simulink model "mavsim_chap8"  (R2015a)
settings: Solver=ode15s  StartTime=0.0  StopTime=80  RelTol=1e-3
InitFcn:
  | param_chap8
undefined symbols (not defined in the file or in its folder): autopilot, drawAircraft, estimate_states, forces_moments, gps, P, plotextramavstatevariables, plotmavstatevariables, sensors, true_states
libraries: simulink x4
settings Model: CovSFcnEnable=off  Creator=beard  LastModifiedBy=Scott
settings DataIOCC: SignalLoggingSaveFormat=ModelDataLogs
settings OptimizationCC: ExpressionDepthLimit=2147483647  InitFltsAndDblsToZero=on
settings DebuggingCC: UnderspecifiedInitializationDetection=Classic  MergeDetectMultiDrivingBlocksExec=none  SolverPrmCheckMsg=warning  FcnCallInpInsideContextMsg=UseLocalSettings  StateNameClashWarn=warning
settings SFSimCC: SimParseCustomCode=off
settings GRTTargetCC: CombineOutputUpdateFcns=off  GRTInterface=on

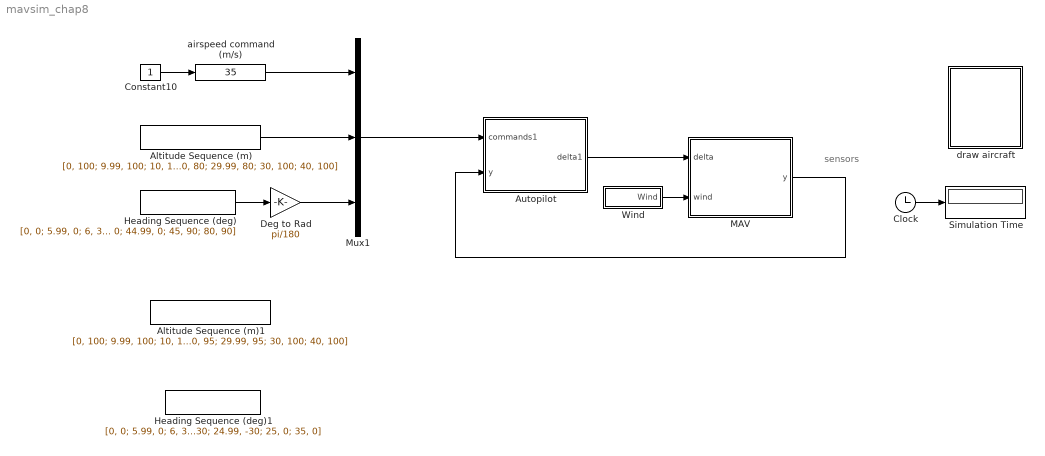
== system mavsim_chap8 ==
  note: sensors
  Altitude Sequence (m) : FromWorkspace  VariableName=[0, 100; 9.99, 100; 10, 120; 19.99, 120; 20, 80; 29.99, 80; 30, 100; 40, 100]  SampleTime=0
  Altitude Sequence (m)1 : FromWorkspace  VariableName=[0, 100; 9.99, 100; 10, 105; 19.99, 105; 20, 95; 29.99, 95; 30, 100; 40, 100]  SampleTime=0
  Autopilot : Subsystem
      mask Display: image(imread('kestrel.jpg'))
  Clock : Clock
  Constant10 : Constant
  Deg to Rad : Gain  Gain=pi/180
  Heading Sequence (deg) : FromWorkspace  VariableName=[0, 0; 5.99, 0; 6, 30; 14.99, 30; 15, -30; 24.99, -30; 25, 0; 35, 0; 44.99, 0; 45, 90; 80, 90]  SampleTime=0
  Heading Sequence (deg)1 : FromWorkspace  VariableName=[0, 0; 5.99, 0; 6, 30; 14.99, 30; 15, -30; 24.99, -30; 25, 0; 35, 0]  SampleTime=0
  MAV : Subsystem
      mask Display: image(imread('batcam.png'))
  Mux1 : Mux  Inputs=3
  Simulation Time : Display
  Wind : Subsystem
  airspeed command (m/s) : simulink/Math Operations/Slider Gain  low=5  gain=35  high=35
  draw aircraft : Subsystem
      mask Display: image(imread('tv.jpg'))
  wires:
  Clock/1 -> Simulation Time/1
  Constant10/1 -> airspeed command (m/s)/1
  airspeed command (m/s)/1 -> Mux1/1
  Mux1/1 -> Autopilot/1(commands1)
  Heading Sequence (deg)/1 -> Deg to Rad/1
  Altitude Sequence (m)/1 -> Mux1/2
  Wind/1(Wind) -> MAV/2(wind)
  Autopilot/1(delta1) -> MAV/1(delta)
  MAV/1(y) -> Autopilot/2(y)
  Deg to Rad/1 -> Mux1/3

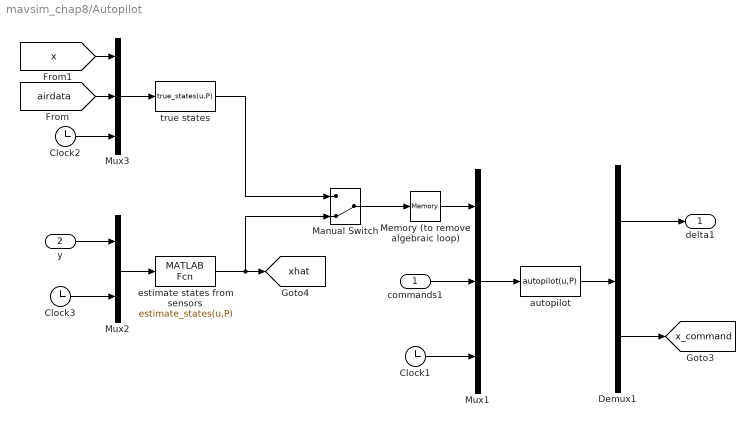
== system mavsim_chap8/Autopilot ==
  commands1 : Inport
  y : Inport  Port=2
  Clock1 : Clock
  Clock2 : Clock
  Clock3 : Clock
  Demux1 : Demux  Outputs=[4;12]
  Manual Switch : ManualSwitch  CurrentSetting=0
  Memory (to remove algebraic loop) : Memory
  Mux1 : Mux  Inputs=3
  Mux2 : Mux  Inputs=2
  Mux3 : Mux  Inputs=3
  autopilot : MATLABFcn  MATLABFcn=autopilot(u,P)  OutputDimensions=4+12  SampleTime=P.Ts
  estimate states from sensors : MATLABFcn  MATLABFcn=estimate_states(u,P)  OutputDimensions=19  SampleTime=P.Ts
  true states : MATLABFcn  MATLABFcn=true_states(u,P)  OutputDimensions=19  SampleTime=P.Ts
  delta1 : Outport
  tag scope: x_command=global, xhat=global
  wires:
  Mux1/1 -> autopilot/1
  autopilot/1 -> Demux1/1
  Demux1/1 -> delta1/1
  Demux1/2 -> [x_command]
  commands1/1 -> Mux1/2
  Mux2/1 -> estimate states from sensors/1
  y/1 -> Mux2/1
  Memory (to remove algebraic loop)/1 -> Mux1/1
  Manual Switch/1 -> Memory (to remove algebraic loop)/1
  true states/1 -> Manual Switch/1
  Mux3/1 -> true states/1
  [airdata] -> Mux3/2
  [x] -> Mux3/1
  Clock1/1 -> Mux1/3
  Clock2/1 -> Mux3/3
  Clock3/1 -> Mux2/2
  estimate states from sensors/1 -> Manual Switch/2, [xhat]

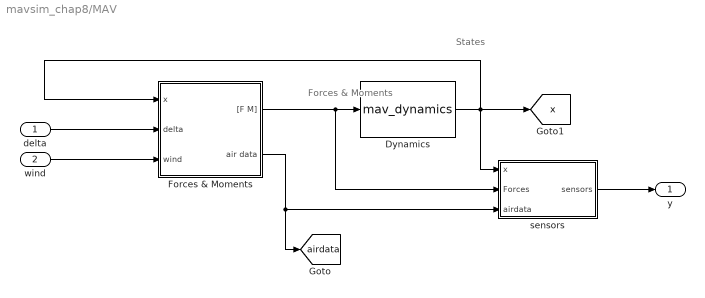
== system mavsim_chap8/MAV ==
  note: States
  note: Forces & Moments
  delta : Inport
  wind : Inport  Port=2
  Dynamics : S-Function  FunctionName=mav_dynamics  Parameters=P
  Forces & Moments : Subsystem
  sensors : Subsystem
  y : Outport
  tag scope: airdata=global, x=global
  wires:
  wind/1 -> Forces & Moments/3(wind)
  delta/1 -> Forces & Moments/2(delta)
  Forces & Moments/2(air data) -> sensors/3(airdata), [airdata]
  Forces & Moments/1("[F M]") -> sensors/2(Forces), Dynamics/1
  Dynamics/1 -> [x], sensors/1(x), Forces & Moments/1(x)
  sensors/1(sensors) -> y/1

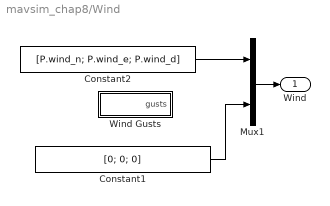
== system mavsim_chap8/Wind ==
  Constant1 : Constant  Value=[0; 0; 0]
  Constant2 : Constant  Value=[P.wind_n; P.wind_e; P.wind_d]
  Mux1 : Mux  Inputs=2
  Wind Gusts : Subsystem
  Wind : Outport
  wires:
  Constant1/1 -> Mux1/2
  Mux1/1 -> Wind/1
  Constant2/1 -> Mux1/1

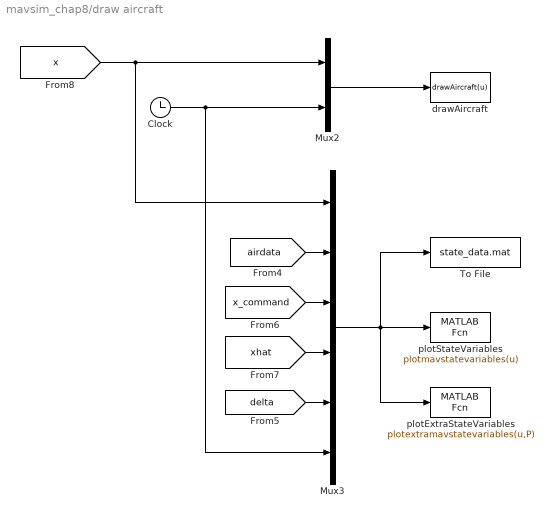
== system mavsim_chap8/draw aircraft ==
  Clock : Clock
  Mux2 : Mux  Inputs=2
  Mux3 : Mux  Inputs=6
  To File : ToFile  Filename=state_data.mat
  drawAircraft : MATLABFcn  MATLABFcn=drawAircraft(u)  OutputDimensions=0  SampleTime=0.1
  plotExtraStateVariables : MATLABFcn  MATLABFcn=plotextramavstatevariables(u,P)  OutputDimensions=0  SampleTime=0.1
  plotStateVariables : MATLABFcn  MATLABFcn=plotmavstatevariables(u)  OutputDimensions=0  SampleTime=0.1
  wires:
  Mux2/1 -> drawAircraft/1
  [x] -> Mux2/1, Mux3/1
  Clock/1 -> Mux2/2, Mux3/6
  Mux3/1 -> plotStateVariables/1, plotExtraStateVariables/1, To File/1
  [xhat] -> Mux3/4
  [x_command] -> Mux3/3
  [delta] -> Mux3/5
  [airdata] -> Mux3/2

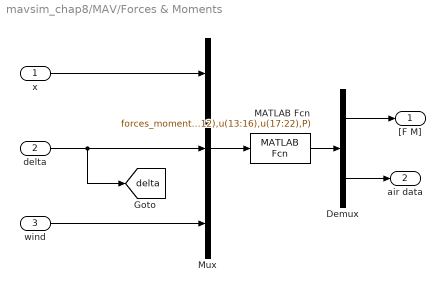
== system mavsim_chap8/MAV/Forces & Moments ==
  x : Inport
  delta : Inport  Port=2
  wind : Inport  Port=3
  Demux : Demux  Outputs=[6;6]
  MATLAB Fcn : MATLABFcn  MATLABFcn=forces_moments(u(1:12),u(13:16),u(17:22),P)  OutputDimensions=12
  Mux : Mux  Inputs=3
  "[F M]" : Outport
  air data : Outport  Port=2
  tag scope: delta=global
  wires:
  Demux/2 -> air data/1
  Mux/1 -> MATLAB Fcn/1
  Demux/1 -> "[F M]"/1
  MATLAB Fcn/1 -> Demux/1
  wind/1 -> Mux/3
  delta/1 -> Mux/2, [delta]
  x/1 -> Mux/1

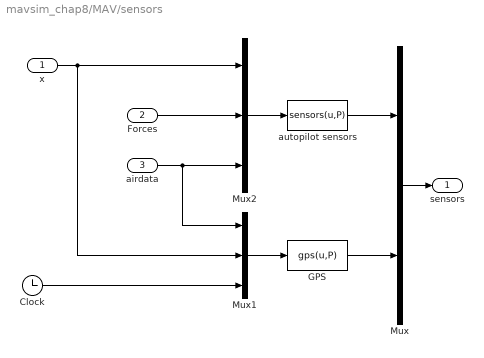
== system mavsim_chap8/MAV/sensors ==
  x : Inport
  Forces : Inport  Port=2
  airdata : Inport  Port=3
  Clock : Clock
  GPS : MATLABFcn  MATLABFcn=gps(u,P)  OutputDimensions=5  SampleTime=P.Ts_gps
  Mux : Mux  Inputs=2
  Mux1 : Mux  Inputs=3
  Mux2 : Mux  Inputs=3
  autopilot sensors : MATLABFcn  MATLABFcn=sensors(u,P)  OutputDimensions=8  SampleTime=P.Ts
  sensors : Outport
  wires:
  x/1 -> Mux1/2, Mux2/1
  Mux/1 -> sensors/1
  airdata/1 -> Mux1/1, Mux2/3
  Forces/1 -> Mux2/2
  Mux2/1 -> autopilot sensors/1
  Clock/1 -> Mux1/3
  Mux1/1 -> GPS/1
  GPS/1 -> Mux/2
  autopilot sensors/1 -> Mux/1

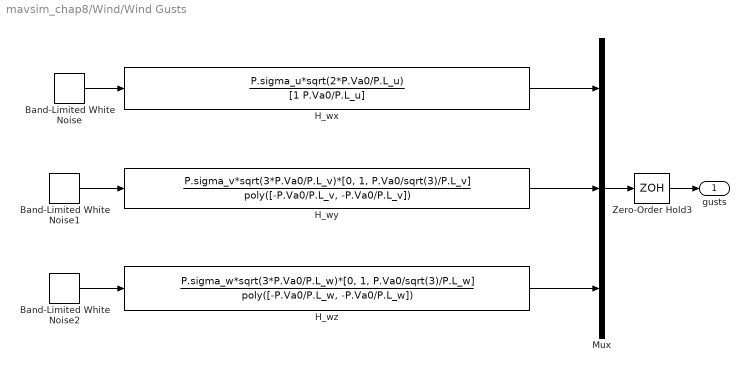
== system mavsim_chap8/Wind/Wind Gusts ==
  Band-Limited White Noise : simulink/Sources/Band-Limited White Noise  Cov=[1]  Ts=P.Ts  seed=[23341]
  Band-Limited White Noise1 : simulink/Sources/Band-Limited White Noise  Cov=[1]  Ts=P.Ts  seed=[23341]
  Band-Limited White Noise2 : simulink/Sources/Band-Limited White Noise  Cov=[1]  Ts=P.Ts  seed=[23341]
  H_wx : TransferFcn  Numerator=P.sigma_u*sqrt(2*P.Va0/P.L_u)  Denominator=[1 P.Va0/P.L_u]
  H_wy : TransferFcn  Numerator=P.sigma_v*sqrt(3*P.Va0/P.L_v)*[0, 1, P.Va0/sqrt(3)/P.L_v]  Denominator=poly([-P.Va0/P.L_v, -P.Va0/P.L_v])
  H_wz : TransferFcn  Numerator=P.sigma_w*sqrt(3*P.Va0/P.L_w)*[0, 1, P.Va0/sqrt(3)/P.L_w]  Denominator=poly([-P.Va0/P.L_w, -P.Va0/P.L_w])
  Mux : Mux  Inputs=3
  Zero-Order Hold3 : ZeroOrderHold  SampleTime=P.Ts
  gusts : Outport
  wires:
  H_wx/1 -> Mux/1
  Band-Limited White Noise/1 -> H_wx/1
  H_wy/1 -> Mux/2
  Band-Limited White Noise1/1 -> H_wy/1
  H_wz/1 -> Mux/3
  Band-Limited White Noise2/1 -> H_wz/1
  Mux/1 -> Zero-Order Hold3/1
  Zero-Order Hold3/1 -> gusts/1
